simulink model "task2cd"  (R2018b)
settings: Solver=VariableStepAuto  StartTime=0.0  StopTime=10.0  RelTol=1e-3
libraries: dspsrcs4 x1
settings Model: Creator=root  LastModifiedBy=root

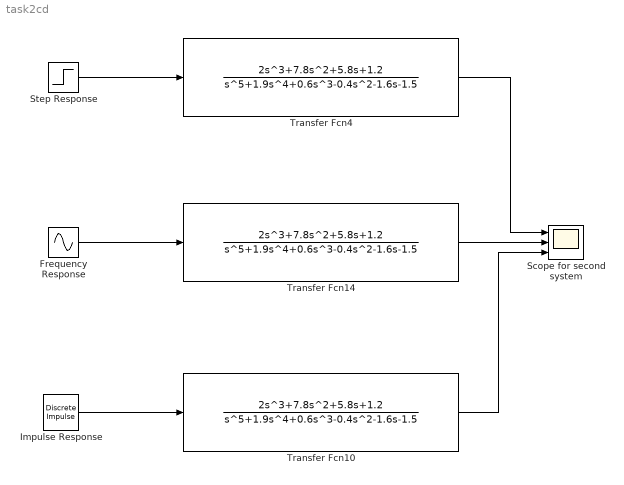
== system task2cd ==
  Frequency Response : Sin  SampleTime=0
  "Impulse Response " : dspsrcs4/Discrete  Impulse  Delay=0  SampleTime=1  FrameSample=1  OutputFrames=off  dataType=double  isSigned=on  wordLen=16  udDataType=sfix(16)  fracBitsMode=Best precision  numFracBits=15  OutDataTypeStr=double  LastOutDataTypeStr=double
  "Scope for second system " : Scope  NumInputPorts=3
  "Step Response " : Step  SampleTime=0
  Transfer Fcn10 : TransferFcn  Numerator=[2 7.8 5.8 1.2]  Denominator=[1 1.9 0.6 -0.4 -1.6 -1.5]
  Transfer Fcn14 : TransferFcn  Numerator=[2 7.8 5.8 1.2]  Denominator=[1 1.9 0.6 -0.4 -1.6 -1.5]
  Transfer Fcn4 : TransferFcn  Numerator=[2 7.8 5.8 1.2]  Denominator=[1 1.9 0.6 -0.4 -1.6 -1.5]
  wires:
  Transfer Fcn4/1 -> "Scope for second system "/1
  "Step Response "/1 -> Transfer Fcn4/1
  Frequency Response/1 -> Transfer Fcn14/1
  Transfer Fcn10/1 -> "Scope for second system "/3
  "Impulse Response "/1 -> Transfer Fcn10/1
  Transfer Fcn14/1 -> "Scope for second system "/2
